simulink model "PLANET_v2"  (R2018b)
settings: Solver=FixedStepAuto  StartTime=0.0  StopTime=span-1  FixedStep=0.1  RelTol=1e-3
undefined symbols (not defined in the file): CHP_eta_el, CHP_eta_th, CHP_Pn, control, dh_demand, DH_elB_Cap, DH_elB_eff, DH_gas_B_Cap, DH_gas_B_eff, DH_HP_Cap, DH_HP_COP, DiscIntNeverNeededParam, dt, h_elD, lhd_demand, LHD_elB_Cap, LHD_elB_eff, LHD_gas_B_Cap, LHD_gas_B_eff, LHD_HP_Cap, LHD_HP_COP, Liion_cap, Liion_charge, Liion_dis, Liion_eff_ch, Liion_eff_dis, PCI, PtG_cap, PtG_eta_elcto, PtG_eta_meth, PtG_eta_th, PVPower, RES_curtailment_on_off, tt, WindPower
libraries: simulink x1
(part 5 of 5)

== system PLANET_v2/Control /Surplus dispacth/4: P2H Li-ion P2G/P2H/HEAT PUMP DH/If Action Subsystem1 ==
  Surplus : Inport
  Heat demand : Inport  Port=2
  Action Port : ActionPort  ActionType=elseif
  COP : Gain  Gain=COP
  Constant : Constant  Value=0
  Sum : Sum  Inputs=-+|
  New surplus : Outport
  New heat demand : Outport  Port=2
  wires:
  Heat demand/1 -> Sum/2
  COP/1 -> Sum/1
  Sum/1 -> New heat demand/1
  Constant/1 -> New surplus/1
  Surplus/1 -> COP/1

== system PLANET_v2/Control /Surplus dispacth/4: P2H Li-ion P2G/P2H/HEAT PUMP DH/If Action Subsystem2 ==
  Surplus : Inport
  Heat demand : Inport  Port=2
  Action Port : ActionPort  ActionType=then
  New surplus : Outport
  New heat demand : Outport  Port=2
  wires:
  Heat demand/1 -> New heat demand/1
  Surplus/1 -> New surplus/1

== system PLANET_v2/Control /Surplus dispacth/4: P2H Li-ion P2G/P2H/HEAT PUMP DH/Max input control ==
  El input : Inport
  Max el input : Inport  Port=2
  If Action Subsystem3 : Subsystem  TreatAsAtomicUnit=on
  If Action Subsystem4 : Subsystem  TreatAsAtomicUnit=on
  If1 : If  NumInputs=2  IfExpression=u1 > u2
  Merge1 : Merge
  Merge2 : Merge
  to PtH : Outport
  Bypassed : Outport  Port=2
  wires:
  If Action Subsystem4/2(to Pth1) -> Merge1/2
  Merge1/1 -> Bypassed/1
  If Action Subsystem4/1(to Pth) -> Merge2/2
  Max el input/1 -> If1/2, If Action Subsystem3/2(Cap)
  If1/2 -> If Action Subsystem4/Action
  If1/1 -> If Action Subsystem3/Action
  El input/1 -> If1/1, If Action Subsystem3/1(Surp), If Action Subsystem4/1(Surplus)
  If Action Subsystem3/2(Bypassed surp) -> Merge1/1
  If Action Subsystem3/1(to PtH) -> Merge2/1
  Merge2/1 -> to PtH/1

== system PLANET_v2/Control /Surplus dispacth/4: P2H Li-ion P2G/P2H/HEAT PUMP local/If Action Subsystem ==
  Surplus : Inport
  Heat demand : Inport  Port=2
  Action Port : ActionPort  ActionType=else
  " " : Gain  Gain=1/COP
  Constant : Constant  Value=0
  Sum : Sum  Inputs=|+-
  New surplus : Outport
  New heat demand : Outport  Port=2
  wires:
  Constant/1 -> New heat demand/1
  Surplus/1 -> Sum/1
  Heat demand/1 -> " "/1
  Sum/1 -> New surplus/1
  " "/1 -> Sum/2

== system PLANET_v2/Control /Surplus dispacth/4: P2H Li-ion P2G/P2H/HEAT PUMP local/If Action Subsystem1 ==
  Surplus : Inport
  Heat demand : Inport  Port=2
  Action Port : ActionPort  ActionType=elseif
  COP : Gain  Gain=COP
  Constant : Constant  Value=0
  Sum : Sum  Inputs=-+|
  New surplus : Outport
  New heat demand : Outport  Port=2
  wires:
  Heat demand/1 -> Sum/2
  COP/1 -> Sum/1
  Sum/1 -> New heat demand/1
  Constant/1 -> New surplus/1
  Surplus/1 -> COP/1

== system PLANET_v2/Control /Surplus dispacth/4: P2H Li-ion P2G/P2H/HEAT PUMP local/If Action Subsystem2 ==
  Surplus : Inport
  Heat demand : Inport  Port=2
  Action Port : ActionPort  ActionType=then
  New surplus : Outport
  New heat demand : Outport  Port=2
  wires:
  Heat demand/1 -> New heat demand/1
  Surplus/1 -> New surplus/1

== system PLANET_v2/Control /Surplus dispacth/4: P2H Li-ion P2G/P2H/HEAT PUMP local/Max input control ==
  El input : Inport
  Max el input : Inport  Port=2
  If Action Subsystem3 : Subsystem  TreatAsAtomicUnit=on
  If Action Subsystem4 : Subsystem  TreatAsAtomicUnit=on
  If1 : If  NumInputs=2  IfExpression=u1 > u2
  Merge1 : Merge
  Merge2 : Merge
  to PtH : Outport
  Bypassed : Outport  Port=2
  wires:
  If Action Subsystem4/2(to Pth1) -> Merge1/2
  Merge1/1 -> Bypassed/1
  If Action Subsystem4/1(to Pth) -> Merge2/2
  Max el input/1 -> If1/2, If Action Subsystem3/2(Cap)
  If1/2 -> If Action Subsystem4/Action
  If1/1 -> If Action Subsystem3/Action
  El input/1 -> If1/1, If Action Subsystem3/1(Surp), If Action Subsystem4/1(Surplus)
  If Action Subsystem3/2(Bypassed surp) -> Merge1/1
  If Action Subsystem3/1(to PtH) -> Merge2/1
  Merge2/1 -> to PtH/1

== system PLANET_v2/Control /Surplus dispacth/5: P2H P2G Li-ion /P2H/Electric boiler DH/If Action Subsystem ==
  Surplus : Inport
  Heat demand : Inport  Port=2
  Action Port : ActionPort  ActionType=else
  " " : Gain  Gain=1/th_eff
  Constant : Constant  Value=0
  Sum : Sum  Inputs=|+-
  New surplus : Outport
  New heat demand : Outport  Port=2
  wires:
  Constant/1 -> New heat demand/1
  Surplus/1 -> Sum/1
  Heat demand/1 -> " "/1
  Sum/1 -> New surplus/1
  " "/1 -> Sum/2

== system PLANET_v2/Control /Surplus dispacth/5: P2H P2G Li-ion /P2H/Electric boiler DH/If Action Subsystem1 ==
  Surplus : Inport
  Heat demand : Inport  Port=2
  Action Port : ActionPort  ActionType=elseif
  Constant : Constant  Value=0
  Sum : Sum  Inputs=-+|
  th_eff : Gain  Gain=th_eff
  New surplus : Outport
  New heat demand : Outport  Port=2
  wires:
  Heat demand/1 -> Sum/2
  th_eff/1 -> Sum/1
  Sum/1 -> New heat demand/1
  Constant/1 -> New surplus/1
  Surplus/1 -> th_eff/1

== system PLANET_v2/Control /Surplus dispacth/5: P2H P2G Li-ion /P2H/Electric boiler DH/If Action Subsystem2 ==
  Surplus : Inport
  Heat demand : Inport  Port=2
  Action Port : ActionPort  ActionType=then
  New surplus : Outport
  New heat demand : Outport  Port=2
  wires:
  Heat demand/1 -> New heat demand/1
  Surplus/1 -> New surplus/1

== system PLANET_v2/Control /Surplus dispacth/5: P2H P2G Li-ion /P2H/Electric boiler DH/Max input control ==
  El input : Inport
  Max el input : Inport  Port=2
  If Action Subsystem3 : Subsystem  TreatAsAtomicUnit=on
  If Action Subsystem4 : Subsystem  TreatAsAtomicUnit=on
  If1 : If  NumInputs=2  IfExpression=u1 > u2
  Merge1 : Merge
  Merge2 : Merge
  to PtH : Outport
  Bypassed : Outport  Port=2
  wires:
  If Action Subsystem4/2(to Pth1) -> Merge1/2
  Merge1/1 -> Bypassed/1
  If Action Subsystem4/1(to Pth) -> Merge2/2
  Max el input/1 -> If1/2, If Action Subsystem3/2(Cap)
  If1/2 -> If Action Subsystem4/Action
  If1/1 -> If Action Subsystem3/Action
  El input/1 -> If1/1, If Action Subsystem3/1(Surp), If Action Subsystem4/1(Surplus)
  If Action Subsystem3/2(Bypassed surp) -> Merge1/1
  If Action Subsystem3/1(to PtH) -> Merge2/1
  Merge2/1 -> to PtH/1

== system PLANET_v2/Control /Surplus dispacth/5: P2H P2G Li-ion /P2H/Electric boiler LHD/If Action Subsystem ==
  Surplus : Inport
  Heat demand : Inport  Port=2
  Action Port : ActionPort  ActionType=else
  " " : Gain  Gain=1/th_eff
  Constant : Constant  Value=0
  Sum : Sum  Inputs=|+-
  New surplus : Outport
  New heat demand : Outport  Port=2
  wires:
  Constant/1 -> New heat demand/1
  Surplus/1 -> Sum/1
  Heat demand/1 -> " "/1
  Sum/1 -> New surplus/1
  " "/1 -> Sum/2

== system PLANET_v2/Control /Surplus dispacth/5: P2H P2G Li-ion /P2H/Electric boiler LHD/If Action Subsystem1 ==
  Surplus : Inport
  Heat demand : Inport  Port=2
  Action Port : ActionPort  ActionType=elseif
  Constant : Constant  Value=0
  Sum : Sum  Inputs=-+|
  th_eff : Gain  Gain=th_eff
  New surplus : Outport
  New heat demand : Outport  Port=2
  wires:
  Heat demand/1 -> Sum/2
  th_eff/1 -> Sum/1
  Sum/1 -> New heat demand/1
  Constant/1 -> New surplus/1
  Surplus/1 -> th_eff/1

== system PLANET_v2/Control /Surplus dispacth/5: P2H P2G Li-ion /P2H/Electric boiler LHD/If Action Subsystem2 ==
  Surplus : Inport
  Heat demand : Inport  Port=2
  Action Port : ActionPort  ActionType=then
  New surplus : Outport
  New heat demand : Outport  Port=2
  wires:
  Heat demand/1 -> New heat demand/1
  Surplus/1 -> New surplus/1

== system PLANET_v2/Control /Surplus dispacth/5: P2H P2G Li-ion /P2H/Electric boiler LHD/Max input control ==
  El input : Inport
  Max el input : Inport  Port=2
  If Action Subsystem3 : Subsystem  TreatAsAtomicUnit=on
  If Action Subsystem4 : Subsystem  TreatAsAtomicUnit=on
  If1 : If  NumInputs=2  IfExpression=u1 > u2
  Merge1 : Merge
  Merge2 : Merge
  to PtH : Outport
  Bypassed : Outport  Port=2
  wires:
  If Action Subsystem4/2(to Pth1) -> Merge1/2
  Merge1/1 -> Bypassed/1
  If Action Subsystem4/1(to Pth) -> Merge2/2
  Max el input/1 -> If1/2, If Action Subsystem3/2(Cap)
  If1/2 -> If Action Subsystem4/Action
  If1/1 -> If Action Subsystem3/Action
  El input/1 -> If1/1, If Action Subsystem3/1(Surp), If Action Subsystem4/1(Surplus)
  If Action Subsystem3/2(Bypassed surp) -> Merge1/1
  If Action Subsystem3/1(to PtH) -> Merge2/1
  Merge2/1 -> to PtH/1

== system PLANET_v2/Control /Surplus dispacth/5: P2H P2G Li-ion /P2H/HEAT PUMP DH/If Action Subsystem ==
  Surplus : Inport
  Heat demand : Inport  Port=2
  Action Port : ActionPort  ActionType=else
  " " : Gain  Gain=1/COP
  Constant : Constant  Value=0
  Sum : Sum  Inputs=|+-
  New surplus : Outport
  New heat demand : Outport  Port=2
  wires:
  Constant/1 -> New heat demand/1
  Surplus/1 -> Sum/1
  Heat demand/1 -> " "/1
  Sum/1 -> New surplus/1
  " "/1 -> Sum/2

== system PLANET_v2/Control /Surplus dispacth/5: P2H P2G Li-ion /P2H/HEAT PUMP DH/If Action Subsystem1 ==
  Surplus : Inport
  Heat demand : Inport  Port=2
  Action Port : ActionPort  ActionType=elseif
  COP : Gain  Gain=COP
  Constant : Constant  Value=0
  Sum : Sum  Inputs=-+|
  New surplus : Outport
  New heat demand : Outport  Port=2
  wires:
  Heat demand/1 -> Sum/2
  COP/1 -> Sum/1
  Sum/1 -> New heat demand/1
  Constant/1 -> New surplus/1
  Surplus/1 -> COP/1

== system PLANET_v2/Control /Surplus dispacth/5: P2H P2G Li-ion /P2H/HEAT PUMP DH/If Action Subsystem2 ==
  Surplus : Inport
  Heat demand : Inport  Port=2
  Action Port : ActionPort  ActionType=then
  New surplus : Outport
  New heat demand : Outport  Port=2
  wires:
  Heat demand/1 -> New heat demand/1
  Surplus/1 -> New surplus/1

== system PLANET_v2/Control /Surplus dispacth/5: P2H P2G Li-ion /P2H/HEAT PUMP DH/Max input control ==
  El input : Inport
  Max el input : Inport  Port=2
  If Action Subsystem3 : Subsystem  TreatAsAtomicUnit=on
  If Action Subsystem4 : Subsystem  TreatAsAtomicUnit=on
  If1 : If  NumInputs=2  IfExpression=u1 > u2
  Merge1 : Merge
  Merge2 : Merge
  to PtH : Outport
  Bypassed : Outport  Port=2
  wires:
  If Action Subsystem4/2(to Pth1) -> Merge1/2
  Merge1/1 -> Bypassed/1
  If Action Subsystem4/1(to Pth) -> Merge2/2
  Max el input/1 -> If1/2, If Action Subsystem3/2(Cap)
  If1/2 -> If Action Subsystem4/Action
  If1/1 -> If Action Subsystem3/Action
  El input/1 -> If1/1, If Action Subsystem3/1(Surp), If Action Subsystem4/1(Surplus)
  If Action Subsystem3/2(Bypassed surp) -> Merge1/1
  If Action Subsystem3/1(to PtH) -> Merge2/1
  Merge2/1 -> to PtH/1

== system PLANET_v2/Control /Surplus dispacth/5: P2H P2G Li-ion /P2H/HEAT PUMP local/If Action Subsystem ==
  Surplus : Inport
  Heat demand : Inport  Port=2
  Action Port : ActionPort  ActionType=else
  " " : Gain  Gain=1/COP
  Constant : Constant  Value=0
  Sum : Sum  Inputs=|+-
  New surplus : Outport
  New heat demand : Outport  Port=2
  wires:
  Constant/1 -> New heat demand/1
  Surplus/1 -> Sum/1
  Heat demand/1 -> " "/1
  Sum/1 -> New surplus/1
  " "/1 -> Sum/2

== system PLANET_v2/Control /Surplus dispacth/5: P2H P2G Li-ion /P2H/HEAT PUMP local/If Action Subsystem1 ==
  Surplus : Inport
  Heat demand : Inport  Port=2
  Action Port : ActionPort  ActionType=elseif
  COP : Gain  Gain=COP
  Constant : Constant  Value=0
  Sum : Sum  Inputs=-+|
  New surplus : Outport
  New heat demand : Outport  Port=2
  wires:
  Heat demand/1 -> Sum/2
  COP/1 -> Sum/1
  Sum/1 -> New heat demand/1
  Constant/1 -> New surplus/1
  Surplus/1 -> COP/1

== system PLANET_v2/Control /Surplus dispacth/5: P2H P2G Li-ion /P2H/HEAT PUMP local/If Action Subsystem2 ==
  Surplus : Inport
  Heat demand : Inport  Port=2
  Action Port : ActionPort  ActionType=then
  New surplus : Outport
  New heat demand : Outport  Port=2
  wires:
  Heat demand/1 -> New heat demand/1
  Surplus/1 -> New surplus/1

== system PLANET_v2/Control /Surplus dispacth/5: P2H P2G Li-ion /P2H/HEAT PUMP local/Max input control ==
  El input : Inport
  Max el input : Inport  Port=2
  If Action Subsystem3 : Subsystem  TreatAsAtomicUnit=on
  If Action Subsystem4 : Subsystem  TreatAsAtomicUnit=on
  If1 : If  NumInputs=2  IfExpression=u1 > u2
  Merge1 : Merge
  Merge2 : Merge
  to PtH : Outport
  Bypassed : Outport  Port=2
  wires:
  If Action Subsystem4/2(to Pth1) -> Merge1/2
  Merge1/1 -> Bypassed/1
  If Action Subsystem4/1(to Pth) -> Merge2/2
  Max el input/1 -> If1/2, If Action Subsystem3/2(Cap)
  If1/2 -> If Action Subsystem4/Action
  If1/1 -> If Action Subsystem3/Action
  El input/1 -> If1/1, If Action Subsystem3/1(Surp), If Action Subsystem4/1(Surplus)
  If Action Subsystem3/2(Bypassed surp) -> Merge1/1
  If Action Subsystem3/1(to PtH) -> Merge2/1
  Merge2/1 -> to PtH/1

== system PLANET_v2/Control /Surplus dispacth/0: Li-ion P2G P2H1/P2H/Electric boiler DH/Max input control/If Action Subsystem3 ==
  Surp : Inport
  Cap : Inport  Port=2
  Action Port : ActionPort  ActionType=then
  Sum : Sum  Inputs=|+-
  to PtH : Outport
  Bypassed surp : Outport  Port=2
  wires:
  Cap/1 -> Sum/2, to PtH/1
  Surp/1 -> Sum/1
  Sum/1 -> Bypassed surp/1

== system PLANET_v2/Control /Surplus dispacth/0: Li-ion P2G P2H1/P2H/Electric boiler DH/Max input control/If Action Subsystem4 ==
  Surplus : Inport
  Action Port : ActionPort  ActionType=else
  Constant : Constant  Value=0
  to Pth : Outport
  to Pth1 : Outport  Port=2
  wires:
  Surplus/1 -> to Pth/1
  Constant/1 -> to Pth1/1

== system PLANET_v2/Control /Surplus dispacth/0: Li-ion P2G P2H1/P2H/Electric boiler LHD/Max input control/If Action Subsystem3 ==
  Surp : Inport
  Cap : Inport  Port=2
  Action Port : ActionPort  ActionType=then
  Sum : Sum  Inputs=|+-
  to PtH : Outport
  Bypassed surp : Outport  Port=2
  wires:
  Cap/1 -> Sum/2, to PtH/1
  Surp/1 -> Sum/1
  Sum/1 -> Bypassed surp/1

== system PLANET_v2/Control /Surplus dispacth/0: Li-ion P2G P2H1/P2H/Electric boiler LHD/Max input control/If Action Subsystem4 ==
  Surplus : Inport
  Action Port : ActionPort  ActionType=else
  Constant : Constant  Value=0
  to Pth : Outport
  to Pth1 : Outport  Port=2
  wires:
  Surplus/1 -> to Pth/1
  Constant/1 -> to Pth1/1

== system PLANET_v2/Control /Surplus dispacth/0: Li-ion P2G P2H1/P2H/HEAT PUMP DH/Max input control/If Action Subsystem3 ==
  Surp : Inport
  Cap : Inport  Port=2
  Action Port : ActionPort  ActionType=then
  Sum : Sum  Inputs=|+-
  to PtH : Outport
  Bypassed surp : Outport  Port=2
  wires:
  Cap/1 -> Sum/2, to PtH/1
  Surp/1 -> Sum/1
  Sum/1 -> Bypassed surp/1

== system PLANET_v2/Control /Surplus dispacth/0: Li-ion P2G P2H1/P2H/HEAT PUMP DH/Max input control/If Action Subsystem4 ==
  Surplus : Inport
  Action Port : ActionPort  ActionType=else
  Constant : Constant  Value=0
  to Pth : Outport
  to Pth1 : Outport  Port=2
  wires:
  Surplus/1 -> to Pth/1
  Constant/1 -> to Pth1/1

== system PLANET_v2/Control /Surplus dispacth/0: Li-ion P2G P2H1/P2H/HEAT PUMP local/Max input control/If Action Subsystem3 ==
  Surp : Inport
  Cap : Inport  Port=2
  Action Port : ActionPort  ActionType=then
  Sum : Sum  Inputs=|+-
  to PtH : Outport
  Bypassed surp : Outport  Port=2
  wires:
  Cap/1 -> Sum/2, to PtH/1
  Surp/1 -> Sum/1
  Sum/1 -> Bypassed surp/1

== system PLANET_v2/Control /Surplus dispacth/0: Li-ion P2G P2H1/P2H/HEAT PUMP local/Max input control/If Action Subsystem4 ==
  Surplus : Inport
  Action Port : ActionPort  ActionType=else
  Constant : Constant  Value=0
  to Pth : Outport
  to Pth1 : Outport  Port=2
  wires:
  Surplus/1 -> to Pth/1
  Constant/1 -> to Pth1/1

== system PLANET_v2/Control /Surplus dispacth/1: Li-ion P2H P2G/P2H/Electric boiler DH/Max input control/If Action Subsystem3 ==
  Surp : Inport
  Cap : Inport  Port=2
  Action Port : ActionPort  ActionType=then
  Sum : Sum  Inputs=|+-
  to PtH : Outport
  Bypassed surp : Outport  Port=2
  wires:
  Sum/1 -> Bypassed surp/1
  Surp/1 -> Sum/1
  Cap/1 -> to PtH/1, Sum/2

== system PLANET_v2/Control /Surplus dispacth/1: Li-ion P2H P2G/P2H/Electric boiler DH/Max input control/If Action Subsystem4 ==
  Surplus : Inport
  Action Port : ActionPort  ActionType=else
  Constant : Constant  Value=0
  to Pth : Outport
  to Pth1 : Outport  Port=2
  wires:
  Constant/1 -> to Pth1/1
  Surplus/1 -> to Pth/1

== system PLANET_v2/Control /Surplus dispacth/1: Li-ion P2H P2G/P2H/Electric boiler LHD/Max input control/If Action Subsystem3 ==
  Surp : Inport
  Cap : Inport  Port=2
  Action Port : ActionPort  ActionType=then
  Sum : Sum  Inputs=|+-
  to PtH : Outport
  Bypassed surp : Outport  Port=2
  wires:
  Sum/1 -> Bypassed surp/1
  Surp/1 -> Sum/1
  Cap/1 -> to PtH/1, Sum/2

== system PLANET_v2/Control /Surplus dispacth/1: Li-ion P2H P2G/P2H/Electric boiler LHD/Max input control/If Action Subsystem4 ==
  Surplus : Inport
  Action Port : ActionPort  ActionType=else
  Constant : Constant  Value=0
  to Pth : Outport
  to Pth1 : Outport  Port=2
  wires:
  Constant/1 -> to Pth1/1
  Surplus/1 -> to Pth/1

== system PLANET_v2/Control /Surplus dispacth/1: Li-ion P2H P2G/P2H/HEAT PUMP DH/Max input control/If Action Subsystem3 ==
  Surp : Inport
  Cap : Inport  Port=2
  Action Port : ActionPort  ActionType=then
  Sum : Sum  Inputs=|+-
  to PtH : Outport
  Bypassed surp : Outport  Port=2
  wires:
  Sum/1 -> Bypassed surp/1
  Surp/1 -> Sum/1
  Cap/1 -> to PtH/1, Sum/2

== system PLANET_v2/Control /Surplus dispacth/1: Li-ion P2H P2G/P2H/HEAT PUMP DH/Max input control/If Action Subsystem4 ==
  Surplus : Inport
  Action Port : ActionPort  ActionType=else
  Constant : Constant  Value=0
  to Pth : Outport
  to Pth1 : Outport  Port=2
  wires:
  Constant/1 -> to Pth1/1
  Surplus/1 -> to Pth/1

== system PLANET_v2/Control /Surplus dispacth/1: Li-ion P2H P2G/P2H/HEAT PUMP local/Max input control/If Action Subsystem3 ==
  Surp : Inport
  Cap : Inport  Port=2
  Action Port : ActionPort  ActionType=then
  Sum : Sum  Inputs=|+-
  to PtH : Outport
  Bypassed surp : Outport  Port=2
  wires:
  Sum/1 -> Bypassed surp/1
  Surp/1 -> Sum/1
  Cap/1 -> to PtH/1, Sum/2

== system PLANET_v2/Control /Surplus dispacth/1: Li-ion P2H P2G/P2H/HEAT PUMP local/Max input control/If Action Subsystem4 ==
  Surplus : Inport
  Action Port : ActionPort  ActionType=else
  Constant : Constant  Value=0
  to Pth : Outport
  to Pth1 : Outport  Port=2
  wires:
  Constant/1 -> to Pth1/1
  Surplus/1 -> to Pth/1

== system PLANET_v2/Control /Surplus dispacth/2: P2G Li-ion P2H/P2H/Electric boiler DH/Max input control/If Action Subsystem3 ==
  Surp : Inport
  Cap : Inport  Port=2
  Action Port : ActionPort  ActionType=then
  Sum : Sum  Inputs=|+-
  to PtH : Outport
  Bypassed surp : Outport  Port=2
  wires:
  Sum/1 -> Bypassed surp/1
  Surp/1 -> Sum/1
  Cap/1 -> to PtH/1, Sum/2

== system PLANET_v2/Control /Surplus dispacth/2: P2G Li-ion P2H/P2H/Electric boiler DH/Max input control/If Action Subsystem4 ==
  Surplus : Inport
  Action Port : ActionPort  ActionType=else
  Constant : Constant  Value=0
  to Pth : Outport
  to Pth1 : Outport  Port=2
  wires:
  Constant/1 -> to Pth1/1
  Surplus/1 -> to Pth/1

== system PLANET_v2/Control /Surplus dispacth/2: P2G Li-ion P2H/P2H/Electric boiler LHD/Max input control/If Action Subsystem3 ==
  Surp : Inport
  Cap : Inport  Port=2
  Action Port : ActionPort  ActionType=then
  Sum : Sum  Inputs=|+-
  to PtH : Outport
  Bypassed surp : Outport  Port=2
  wires:
  Sum/1 -> Bypassed surp/1
  Surp/1 -> Sum/1
  Cap/1 -> to PtH/1, Sum/2

== system PLANET_v2/Control /Surplus dispacth/2: P2G Li-ion P2H/P2H/Electric boiler LHD/Max input control/If Action Subsystem4 ==
  Surplus : Inport
  Action Port : ActionPort  ActionType=else
  Constant : Constant  Value=0
  to Pth : Outport
  to Pth1 : Outport  Port=2
  wires:
  Constant/1 -> to Pth1/1
  Surplus/1 -> to Pth/1

== system PLANET_v2/Control /Surplus dispacth/2: P2G Li-ion P2H/P2H/HEAT PUMP DH/Max input control/If Action Subsystem3 ==
  Surp : Inport
  Cap : Inport  Port=2
  Action Port : ActionPort  ActionType=then
  Sum : Sum  Inputs=|+-
  to PtH : Outport
  Bypassed surp : Outport  Port=2
  wires:
  Sum/1 -> Bypassed surp/1
  Surp/1 -> Sum/1
  Cap/1 -> to PtH/1, Sum/2

== system PLANET_v2/Control /Surplus dispacth/2: P2G Li-ion P2H/P2H/HEAT PUMP DH/Max input control/If Action Subsystem4 ==
  Surplus : Inport
  Action Port : ActionPort  ActionType=else
  Constant : Constant  Value=0
  to Pth : Outport
  to Pth1 : Outport  Port=2
  wires:
  Constant/1 -> to Pth1/1
  Surplus/1 -> to Pth/1

== system PLANET_v2/Control /Surplus dispacth/2: P2G Li-ion P2H/P2H/HEAT PUMP local/Max input control/If Action Subsystem3 ==
  Surp : Inport
  Cap : Inport  Port=2
  Action Port : ActionPort  ActionType=then
  Sum : Sum  Inputs=|+-
  to PtH : Outport
  Bypassed surp : Outport  Port=2
  wires:
  Sum/1 -> Bypassed surp/1
  Surp/1 -> Sum/1
  Cap/1 -> to PtH/1, Sum/2

== system PLANET_v2/Control /Surplus dispacth/2: P2G Li-ion P2H/P2H/HEAT PUMP local/Max input control/If Action Subsystem4 ==
  Surplus : Inport
  Action Port : ActionPort  ActionType=else
  Constant : Constant  Value=0
  to Pth : Outport
  to Pth1 : Outport  Port=2
  wires:
  Constant/1 -> to Pth1/1
  Surplus/1 -> to Pth/1

== system PLANET_v2/Control /Surplus dispacth/3: P2G P2H Li-ion/P2H/Electric boiler DH/Max input control/If Action Subsystem3 ==
  Surp : Inport
  Cap : Inport  Port=2
  Action Port : ActionPort  ActionType=then
  Sum : Sum  Inputs=|+-
  to PtH : Outport
  Bypassed surp : Outport  Port=2
  wires:
  Sum/1 -> Bypassed surp/1
  Surp/1 -> Sum/1
  Cap/1 -> to PtH/1, Sum/2

== system PLANET_v2/Control /Surplus dispacth/3: P2G P2H Li-ion/P2H/Electric boiler DH/Max input control/If Action Subsystem4 ==
  Surplus : Inport
  Action Port : ActionPort  ActionType=else
  Constant : Constant  Value=0
  to Pth : Outport
  to Pth1 : Outport  Port=2
  wires:
  Constant/1 -> to Pth1/1
  Surplus/1 -> to Pth/1

== system PLANET_v2/Control /Surplus dispacth/3: P2G P2H Li-ion/P2H/Electric boiler LHD/Max input control/If Action Subsystem3 ==
  Surp : Inport
  Cap : Inport  Port=2
  Action Port : ActionPort  ActionType=then
  Sum : Sum  Inputs=|+-
  to PtH : Outport
  Bypassed surp : Outport  Port=2
  wires:
  Sum/1 -> Bypassed surp/1
  Surp/1 -> Sum/1
  Cap/1 -> to PtH/1, Sum/2

== system PLANET_v2/Control /Surplus dispacth/3: P2G P2H Li-ion/P2H/Electric boiler LHD/Max input control/If Action Subsystem4 ==
  Surplus : Inport
  Action Port : ActionPort  ActionType=else
  Constant : Constant  Value=0
  to Pth : Outport
  to Pth1 : Outport  Port=2
  wires:
  Constant/1 -> to Pth1/1
  Surplus/1 -> to Pth/1

== system PLANET_v2/Control /Surplus dispacth/3: P2G P2H Li-ion/P2H/HEAT PUMP DH/Max input control/If Action Subsystem3 ==
  Surp : Inport
  Cap : Inport  Port=2
  Action Port : ActionPort  ActionType=then
  Sum : Sum  Inputs=|+-
  to PtH : Outport
  Bypassed surp : Outport  Port=2
  wires:
  Sum/1 -> Bypassed surp/1
  Surp/1 -> Sum/1
  Cap/1 -> to PtH/1, Sum/2

== system PLANET_v2/Control /Surplus dispacth/3: P2G P2H Li-ion/P2H/HEAT PUMP DH/Max input control/If Action Subsystem4 ==
  Surplus : Inport
  Action Port : ActionPort  ActionType=else
  Constant : Constant  Value=0
  to Pth : Outport
  to Pth1 : Outport  Port=2
  wires:
  Constant/1 -> to Pth1/1
  Surplus/1 -> to Pth/1

== system PLANET_v2/Control /Surplus dispacth/3: P2G P2H Li-ion/P2H/HEAT PUMP local/Max input control/If Action Subsystem3 ==
  Surp : Inport
  Cap : Inport  Port=2
  Action Port : ActionPort  ActionType=then
  Sum : Sum  Inputs=|+-
  to PtH : Outport
  Bypassed surp : Outport  Port=2
  wires:
  Sum/1 -> Bypassed surp/1
  Surp/1 -> Sum/1
  Cap/1 -> to PtH/1, Sum/2

== system PLANET_v2/Control /Surplus dispacth/3: P2G P2H Li-ion/P2H/HEAT PUMP local/Max input control/If Action Subsystem4 ==
  Surplus : Inport
  Action Port : ActionPort  ActionType=else
  Constant : Constant  Value=0
  to Pth : Outport
  to Pth1 : Outport  Port=2
  wires:
  Constant/1 -> to Pth1/1
  Surplus/1 -> to Pth/1

== system PLANET_v2/Control /Surplus dispacth/4: P2H Li-ion P2G/P2H/Electric boiler DH/Max input control/If Action Subsystem3 ==
  Surp : Inport
  Cap : Inport  Port=2
  Action Port : ActionPort  ActionType=then
  Sum : Sum  Inputs=|+-
  to PtH : Outport
  Bypassed surp : Outport  Port=2
  wires:
  Sum/1 -> Bypassed surp/1
  Surp/1 -> Sum/1
  Cap/1 -> to PtH/1, Sum/2

== system PLANET_v2/Control /Surplus dispacth/4: P2H Li-ion P2G/P2H/Electric boiler DH/Max input control/If Action Subsystem4 ==
  Surplus : Inport
  Action Port : ActionPort  ActionType=else
  Constant : Constant  Value=0
  to Pth : Outport
  to Pth1 : Outport  Port=2
  wires:
  Constant/1 -> to Pth1/1
  Surplus/1 -> to Pth/1

== system PLANET_v2/Control /Surplus dispacth/4: P2H Li-ion P2G/P2H/Electric boiler LHD/Max input control/If Action Subsystem3 ==
  Surp : Inport
  Cap : Inport  Port=2
  Action Port : ActionPort  ActionType=then
  Sum : Sum  Inputs=|+-
  to PtH : Outport
  Bypassed surp : Outport  Port=2
  wires:
  Sum/1 -> Bypassed surp/1
  Surp/1 -> Sum/1
  Cap/1 -> to PtH/1, Sum/2

== system PLANET_v2/Control /Surplus dispacth/4: P2H Li-ion P2G/P2H/Electric boiler LHD/Max input control/If Action Subsystem4 ==
  Surplus : Inport
  Action Port : ActionPort  ActionType=else
  Constant : Constant  Value=0
  to Pth : Outport
  to Pth1 : Outport  Port=2
  wires:
  Constant/1 -> to Pth1/1
  Surplus/1 -> to Pth/1

== system PLANET_v2/Control /Surplus dispacth/4: P2H Li-ion P2G/P2H/HEAT PUMP DH/Max input control/If Action Subsystem3 ==
  Surp : Inport
  Cap : Inport  Port=2
  Action Port : ActionPort  ActionType=then
  Sum : Sum  Inputs=|+-
  to PtH : Outport
  Bypassed surp : Outport  Port=2
  wires:
  Sum/1 -> Bypassed surp/1
  Surp/1 -> Sum/1
  Cap/1 -> to PtH/1, Sum/2

== system PLANET_v2/Control /Surplus dispacth/4: P2H Li-ion P2G/P2H/HEAT PUMP DH/Max input control/If Action Subsystem4 ==
  Surplus : Inport
  Action Port : ActionPort  ActionType=else
  Constant : Constant  Value=0
  to Pth : Outport
  to Pth1 : Outport  Port=2
  wires:
  Constant/1 -> to Pth1/1
  Surplus/1 -> to Pth/1

== system PLANET_v2/Control /Surplus dispacth/4: P2H Li-ion P2G/P2H/HEAT PUMP local/Max input control/If Action Subsystem3 ==
  Surp : Inport
  Cap : Inport  Port=2
  Action Port : ActionPort  ActionType=then
  Sum : Sum  Inputs=|+-
  to PtH : Outport
  Bypassed surp : Outport  Port=2
  wires:
  Sum/1 -> Bypassed surp/1
  Surp/1 -> Sum/1
  Cap/1 -> to PtH/1, Sum/2

== system PLANET_v2/Control /Surplus dispacth/4: P2H Li-ion P2G/P2H/HEAT PUMP local/Max input control/If Action Subsystem4 ==
  Surplus : Inport
  Action Port : ActionPort  ActionType=else
  Constant : Constant  Value=0
  to Pth : Outport
  to Pth1 : Outport  Port=2
  wires:
  Constant/1 -> to Pth1/1
  Surplus/1 -> to Pth/1

== system PLANET_v2/Control /Surplus dispacth/5: P2H P2G Li-ion /P2H/Electric boiler DH/Max input control/If Action Subsystem3 ==
  Surp : Inport
  Cap : Inport  Port=2
  Action Port : ActionPort  ActionType=then
  Sum : Sum  Inputs=|+-
  to PtH : Outport
  Bypassed surp : Outport  Port=2
  wires:
  Sum/1 -> Bypassed surp/1
  Surp/1 -> Sum/1
  Cap/1 -> to PtH/1, Sum/2

== system PLANET_v2/Control /Surplus dispacth/5: P2H P2G Li-ion /P2H/Electric boiler DH/Max input control/If Action Subsystem4 ==
  Surplus : Inport
  Action Port : ActionPort  ActionType=else
  Constant : Constant  Value=0
  to Pth : Outport
  to Pth1 : Outport  Port=2
  wires:
  Constant/1 -> to Pth1/1
  Surplus/1 -> to Pth/1

== system PLANET_v2/Control /Surplus dispacth/5: P2H P2G Li-ion /P2H/Electric boiler LHD/Max input control/If Action Subsystem3 ==
  Surp : Inport
  Cap : Inport  Port=2
  Action Port : ActionPort  ActionType=then
  Sum : Sum  Inputs=|+-
  to PtH : Outport
  Bypassed surp : Outport  Port=2
  wires:
  Sum/1 -> Bypassed surp/1
  Surp/1 -> Sum/1
  Cap/1 -> to PtH/1, Sum/2

== system PLANET_v2/Control /Surplus dispacth/5: P2H P2G Li-ion /P2H/Electric boiler LHD/Max input control/If Action Subsystem4 ==
  Surplus : Inport
  Action Port : ActionPort  ActionType=else
  Constant : Constant  Value=0
  to Pth : Outport
  to Pth1 : Outport  Port=2
  wires:
  Constant/1 -> to Pth1/1
  Surplus/1 -> to Pth/1

== system PLANET_v2/Control /Surplus dispacth/5: P2H P2G Li-ion /P2H/HEAT PUMP DH/Max input control/If Action Subsystem3 ==
  Surp : Inport
  Cap : Inport  Port=2
  Action Port : ActionPort  ActionType=then
  Sum : Sum  Inputs=|+-
  to PtH : Outport
  Bypassed surp : Outport  Port=2
  wires:
  Sum/1 -> Bypassed surp/1
  Surp/1 -> Sum/1
  Cap/1 -> to PtH/1, Sum/2

== system PLANET_v2/Control /Surplus dispacth/5: P2H P2G Li-ion /P2H/HEAT PUMP DH/Max input control/If Action Subsystem4 ==
  Surplus : Inport
  Action Port : ActionPort  ActionType=else
  Constant : Constant  Value=0
  to Pth : Outport
  to Pth1 : Outport  Port=2
  wires:
  Constant/1 -> to Pth1/1
  Surplus/1 -> to Pth/1

== system PLANET_v2/Control /Surplus dispacth/5: P2H P2G Li-ion /P2H/HEAT PUMP local/Max input control/If Action Subsystem3 ==
  Surp : Inport
  Cap : Inport  Port=2
  Action Port : ActionPort  ActionType=then
  Sum : Sum  Inputs=|+-
  to PtH : Outport
  Bypassed surp : Outport  Port=2
  wires:
  Sum/1 -> Bypassed surp/1
  Surp/1 -> Sum/1
  Cap/1 -> to PtH/1, Sum/2

== system PLANET_v2/Control /Surplus dispacth/5: P2H P2G Li-ion /P2H/HEAT PUMP local/Max input control/If Action Subsystem4 ==
  Surplus : Inport
  Action Port : ActionPort  ActionType=else
  Constant : Constant  Value=0
  to Pth : Outport
  to Pth1 : Outport  Port=2
  wires:
  Constant/1 -> to Pth1/1
  Surplus/1 -> to Pth/1
